simulink model "gssiso"  (Simulink 2.20)
settings: Solver=ode45  StartTime=0.0  StopTime=20.0  MaxStep=0.1  RelTol=1e-3  AbsTol=1e-6
libraries: NelinSys x2
settings Model: ConsistencyChecking=off  RTWPlaceOutputsASAP=off

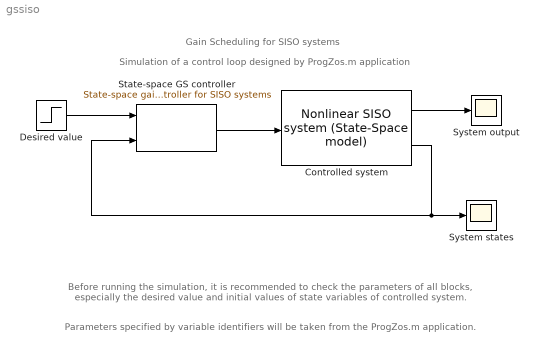
== system gssiso ==
  note: Gain Scheduling for SISO systems
  note: Simulation of a control loop designed by ProgZos.m application
  note: Before running the simulation, it is recommended to check the parameters of all blocks,
      | especially the desired value and initial values of state variables of controlled system.
  note: Parameters specified by variable identifiers will be taken from the ProgZos.m application.
  Controlled system : NelinSys/Nonlinear Systems Synthesis/Nonlinear SISO system (State-Space model)  n=n  Fp=F  Gp=G  Hp=H  pp=[0.1; 0.01]
  Desired value : Step  Time=5  Before=2  After=10
  State-space GS controller : NelinSys/Nonlinear Systems Synthesis/Gain Scheduling Blocks/State-space gain-scheduling controller for SISO systems  n=n  vzorecP=u
  System output : Scope
      settings: TickLabels=on  TimeRange=auto  YMin=-5  YMax=5  SaveToWorkspace=off  SaveName=ScopeData
  System states : Scope
      settings: TickLabels=on  TimeRange=auto  YMin=-5  YMax=5  SaveToWorkspace=off  SaveName=ScopeData
  wires:
  State-space GS controller/1 -> Controlled system/1
  Controlled system/1 -> System output/1
  Controlled system/2 -> State-space GS controller/2, System states/1
  Desired value/1 -> State-space GS controller/1
